simulink model "Tractor_Semitrailer_2023a"  (R2023a)
settings: Solver=VariableStepAuto  StartTime=0.0  StopTime=tmax  FixedStep=dt  RelTol=1e-3  EnableMultiTasking=on
PreLoadFcn:
  | init_vehicle
  | SIMSCAPE_BE_driveline_etrailer_parameters
StartFcn:
  | tic
StopFcn:
  | toc
  | sim_stop_function
undefined symbols (not defined in the file): brake_input, chassis_length, end_val, final_x, final_y, Floor, front_overhang, InputSwitch, L_0f, LD, mass_trailer, massload, pose_t0, sp_t, steer_input, steer_path, steer_ratio, steer_sens, throttle_input, tire_param_drive, tire_param_steer, tire_param_trailer, tire_width, v_0, Vx, wheelbase, X, Y, Z
libraries: sm_lib x367, nesl_utility x273, CommercialVehicleLibrary2G x2, robotalgslib x1, simulink_extras x1
(part 8 of 11)

== system Tractor_Semitrailer_2023a/Tractor_semitrailer /Driver/Control/Simulation end module ==
  x : Inport
  y : Inport  Port=2
  Cast To Boolean : DataTypeConversion  OutDataTypeStr=boolean  SaturateOnIntegerOverflow=off  RndMeth=Floor
  Constant : Constant  Commented=on  Value=end_val
  Constant1 : Constant  Commented=on  Value=end_val
  Constant2 : Constant  Commented=on  Value=v_0
  Constant3 : Constant  Value=final_x
  Constant4 : Constant  Value=final_y
  Constant5 : Constant  Value=0.5
  GreaterThan : RelationalOperator  Commented=on  Operator=<  OutDataTypeStr=boolean  RndMeth=Simplest  InputSameDT=off
  GreaterThan1 : RelationalOperator  Commented=on  Operator=<  OutDataTypeStr=boolean  RndMeth=Simplest  InputSameDT=off
  Less Than : RelationalOperator  Operator=<  OutDataTypeStr=boolean  RndMeth=Simplest  InputSameDT=off
  Scope : Scope
  Sign : Signum  Commented=on
  Sqrt : Sqrt
  Square : Math  Operator=square
  Square1 : Math  Operator=square
  Stop Simulation : Stop  Commented=on
  Stop Simulation1 : Stop
  Sum : Sum
  Sum1 : Sum  Inputs=+-
  Sum2 : Sum  Inputs=+-
  Switch : Switch  Commented=on  Criteria=u2 > Threshold  SaturateOnIntegerOverflow=off  InputSameDT=off
  wires:
  Constant5/1 -> Less Than/2
  Sqrt/1 -> Less Than/1, Scope/1
  Constant4/1 -> Sum2/2
  Sum2/1 -> Square1/1
  Sum1/1 -> Square/1
  Constant3/1 -> Sum1/2
  Sum/1 -> Sqrt/1
  Square1/1 -> Sum/2
  Square/1 -> Sum/1
  Constant/1 -> GreaterThan/2
  x/1 -> Sum1/1
  y/1 -> Sum2/1
  Constant1/1 -> GreaterThan1/2
  Switch/1 -> Stop Simulation/1
  Sign/1 -> Switch/2
  GreaterThan/1 -> Switch/1
  GreaterThan1/1 -> Switch/3
  Constant2/1 -> Sign/1
  Less Than/1 -> Cast To Boolean/1
  Cast To Boolean/1 -> Stop Simulation1/1

== system Tractor_Semitrailer_2023a/Tractor_semitrailer /Semitrailer/Trailer axle 1/Brake//Wheel_bearing ==
  Mdrive : Inport
  Mbrake : Inport  Port=2
  Look-Up Table : Lookup  InputValues=[-5:0.05:5]  Table=-tanh(2*[-5:0.05:5])
  Product1 : Product  InputSameDT=on  SaturateOnIntegerOverflow=on  OutDataTypeStr=Inherit: Same as first input
  Rotational joint around y axis : Subsystem
  Sum : Sum  Inputs=++|
  axle : PMIOPort  Side=Left
  wheel : PMIOPort  Port=2  Side=Right
  omega : Outport  VectorParamsAs1DForOutWhenUnconnected=off
  wires:
  Mbrake/1 -> Product1/1
  Look-Up Table/1 -> Product1/2
  Product1/1 -> Sum/2
  Mdrive/1 -> Sum/1
  Rotational joint around y axis/1(Rotational speed) -> omega/1, Look-Up Table/1
  Sum/1 -> Rotational joint around y axis/1(Torque)
  connections:
  Rotational joint around y axis/LConn1 -- axle/RConn1
  wheel/RConn1 -- Rotational joint around y axis/RConn1

== system Tractor_Semitrailer_2023a/Tractor_semitrailer /Semitrailer/Trailer axle 1/Brake//Wheel_bearing1 ==
  Mdrive : Inport
  Mbrake : Inport  Port=2
  Look-Up Table : Lookup  InputValues=[-5:0.05:5]  Table=-tanh(2*[-5:0.05:5])
  Product1 : Product  InputSameDT=on  SaturateOnIntegerOverflow=on  OutDataTypeStr=Inherit: Same as first input
  Rotational joint around y axis : Subsystem
  Sum : Sum  Inputs=++|
  axle : PMIOPort  Side=Left
  wheel : PMIOPort  Port=2  Side=Right
  omega : Outport  VectorParamsAs1DForOutWhenUnconnected=off
  wires:
  Mbrake/1 -> Product1/1
  Look-Up Table/1 -> Product1/2
  Product1/1 -> Sum/2
  Mdrive/1 -> Sum/1
  Rotational joint around y axis/1(Rotational speed) -> omega/1, Look-Up Table/1
  Sum/1 -> Rotational joint around y axis/1(Torque)
  connections:
  Rotational joint around y axis/LConn1 -- axle/RConn1
  wheel/RConn1 -- Rotational joint around y axis/RConn1

== system Tractor_Semitrailer_2023a/Tractor_semitrailer /Semitrailer/Trailer axle 1/Wheel FL ==
  Bus Creator : BusCreator  Inputs=6
  Bus Creator2 : BusCreator  Inputs=3
  Demux : Demux  Outputs=3
  Demux1 : Demux  Outputs=3
  Geometry Transform : sm_lib/Frames and Transforms/Rigid Transform  TranslationMethod=None  TranslationStandardOffset=0  TranslationStandardOffsetUnits=m  TranslationStandardAxis=+Y  TranslationCartesianOffset=[0 0 0]  TranslationCartesianOffsetUnits=m  TranslationROffset=0  TranslationROffsetUnits=m  TranslationZOffset=0  TranslationZOffsetUnits=m  TranslationThetaOffset=0  TranslationThetaOffsetUnits=deg  RotationMethod=StandardAxis  RotationAngleUnits=deg  RotationStandardAxis=+Z  RotationAngle=sideR*90  RotationArbitraryAxis=[0 0 1]  FollAlignAxisA=+X  BaseAlignAxisA=+Y  FollAlignAxisB=+Y  BaseAlignAxisB=+Z  RotationSequenceAxes=FollowerAxes  RotationSequence=XYX  RotationSequenceAngles=[0 0 0]  RotationSequenceAnglesUnits=deg  RotationMatrix=[1 0 0; 0 1 0; 0 0 1]  Quaternion=[1 0 0 0]
  Inertia : sm_lib/Body Elements/Inertia  InertiaType=Custom  Mass=wheelbody_mass  MassUnits=kg  CenterOfMass=[0 0 0]  CenterOfMassUnits=m  MomentsOfInertia=[Imat(1,1) Imat(2,2) Imat(3,3)]  MomentsOfInertiaUnits=kg*m^2  ProductsOfInertia=[0 0 0]  ProductsOfInertiaUnits=kg*m^2  GraphicType=None  MarkerShape=Inertia  MarkerSize=20  GraphicVisPropType=SimpleVisualProperties  GraphicDiffuseColor=[0.5 0.5 0.5]  GraphicSpecularColor=[0.5 0.5 0.5 1.0]  GraphicAmbientColor=[0.15 0.15 0.15 1.0]  GraphicEmissiveColor=[0.0 0.0 0.0 1.0]  GraphicShininess=75  GraphicOpacity=1.0
  MF Tire FL : sm_lib/Forces and Torques/Magic Formula Tire Force and Torque  TireSide=Left  TireParameters=tire_param  SlipMode=Combined  NumericParameters=[0.1 0.1 0.1 0.1 5.0 1e-4 1e-4 1e-7 1e-7 1e-4 1e-4 0.1 1e-4 1e-4 1e-4 1e-4 1e-4 1e-4 1e-4 1e-4 1e-4]  ScalingCoefficientLMUXMode=FromTireParameters  ScalingCoefficientLMUYMode=FromTireParameters  TireWrenchFrame=ContactFrame  SenseTireForce=on  SenseTireTorque=on  SensePneumaticTrail=off  SenseLongitudinalSlip=off  SenseSaturatedLongitudinalSlip=off  SenseSlipAngle=off  SenseSaturatedSlipAngle=off  SenseTurnSlip=off  SenseRelativeLongitudinalVelocity=off  SenseRelativeLateralVelocity=off  SenseLongitudinalSlipVelocity=off  SenseLateralSlipVelocity=off  SenseYawVelocity=off  SenseCamberAngle=off  SenseSaturatedCamberAngle=off  SenseCamberVelocity=off  SenseSpinVelocity=off  SenseFreeRadius=off  SenseLoadedRadius=off  SenseEffectiveRollingRadius=off  SenseLongitudinalFrictionCoefficient=off  SenseLateralFrictionCoefficient=off  SenseContactBaseRotation=off  SenseContactBaseTranslation=off  SenseContactFollowerRotation=off  SenseContactFollowerTranslation=off
  PS-Simulink Converter : nesl_utility/PS-Simulink Converter  PhysicalDomain=network_engine_domain  SubClassName=ps_output  LeftPortType=input  RightPortType=output  PseudoPeriodic=off  Frequencies=[]  VectorFormat=inherit  Unit=inherit  AffineConversion=off
  PS-Simulink Converter1 : nesl_utility/PS-Simulink Converter  PhysicalDomain=network_engine_domain  SubClassName=ps_output  LeftPortType=input  RightPortType=output  PseudoPeriodic=off  Frequencies=[]  VectorFormat=inherit  Unit=inherit  AffineConversion=off
  PS-Simulink Converter{2..11} (10 alike) : nesl_utility/PS-Simulink Converter  PhysicalDomain=network_engine_domain  SubClassName=ps_output  LeftPortType=input  RightPortType=output  PseudoPeriodic=off  Frequencies=[]  VectorFormat=1-D array  Unit=1  AffineConversion=off
  Reshape : Reshape
  Rigid Transform : sm_lib/Frames and Transforms/Rigid Transform  TranslationMethod=StandardAxis  TranslationStandardOffset=tire_width/2  TranslationStandardOffsetUnits=m  TranslationStandardAxis=+Z  TranslationCartesianOffset=[0 0 0]  TranslationCartesianOffsetUnits=m  TranslationROffset=0  TranslationROffsetUnits=m  TranslationZOffset=0  TranslationZOffsetUnits=m  TranslationThetaOffset=0  TranslationThetaOffsetUnits=deg  RotationMethod=None  RotationAngleUnits=deg  RotationStandardAxis=+Z  RotationAngle=0.0  RotationArbitraryAxis=[0 0 1]  FollAlignAxisA=+X  BaseAlignAxisA=+Y  FollAlignAxisB=+Y  BaseAlignAxisB=+Z  RotationSequenceAxes=FollowerAxes  RotationSequence=XYX  RotationSequenceAngles=[0 0 0]  RotationSequenceAnglesUnits=deg  RotationMatrix=[1 0 0; 0 1 0; 0 0 1]  Quaternion=[1 0 0 0]
  Rim+Tire : sm_lib/Body Elements/File Solid  ExtGeomFileName=wheel.STP  UnitType=Custom  ExtGeomFileUnits=mm  StepReaderType=HEX  ExportConvexHullGeometry=off  InertiaType=Custom  Mass=0  MassUnits=kg  CenterOfMass=[0 0 0]  CenterOfMassUnits=m  MomentsOfInertia=[0 0 0]  MomentsOfInertiaUnits=kg*m^2  ProductsOfInertia=[0 0 0]  ProductsOfInertiaUnits=kg*m^2  BasedOnType=Density  Density=1000  DensityUnits=kg/(m^3)  DoExposeReferenceFrame=on  SerializedFrames=<Frames/>  GraphicType=FromGeometry  MarkerShape=Sphere  MarkerSize=10  GraphicVisPropType=SimpleVisualProperties  GraphicDiffuseColor=[0.8 0.8 0.8]  GraphicSpecularColor=[0.5 0.5 0.5 1.0]  GraphicAmbientColor=[0.15 0.15 0.15 1.0]  GraphicEmissiveColor=[0.0 0.0 0.0 1.0]  GraphicShininess=75  GraphicOpacity=1.0
  Rotation Axis Transform : sm_lib/Frames and Transforms/Rigid Transform  TranslationMethod=None  TranslationStandardOffset=0  TranslationStandardOffsetUnits=m  TranslationStandardAxis=+Z  TranslationCartesianOffset=[0 0 0]  TranslationCartesianOffsetUnits=m  TranslationROffset=0  TranslationROffsetUnits=m  TranslationZOffset=0  TranslationZOffsetUnits=m  TranslationThetaOffset=0  TranslationThetaOffsetUnits=deg  RotationMethod=AlignedAxes  RotationAngleUnits=deg  RotationStandardAxis=-X  RotationAngle=0  RotationArbitraryAxis=[0 0 1]  FollAlignAxisA=+X  BaseAlignAxisA=+X  FollAlignAxisB=+Z  BaseAlignAxisB=+Y  RotationSequenceAxes=FollowerAxes  RotationSequence=XYX  RotationSequenceAngles=[0 0 0]  RotationSequenceAnglesUnits=deg  RotationMatrix=[1 0 0; 0 1 0; 0 0 1]  Quaternion=[1 0 0 0]
  Terminator{,1..6} (7 alike) : Terminator
  Transform Sensor-LocalBodyCS : sm_lib/Frames and Transforms/Transform Sensor  MeasurementFrame=NonRotatingFollower  RotationSequence=XYX  SenseAngle=off  SenseAxis=off  SenseQ=off  SenseR=off  SenseRotationSequence=off  SenseOmegaX=on  SenseOmegaY=on  SenseOmegaZ=on  SenseQDot=off  SenseRDot=off  SenseRotationSequenceDot=off  SenseAlphaX=off  SenseAlphaY=off  SenseAlphaZ=off  SenseQDDot=off  SenseRDDot=off  SenseX=off  SenseY=off  SenseZ=off  SenseRad=off  SenseAzim=off  SenseDist=off  SenseInc=off  SenseXDot=on  SenseYDot=on  SenseZDot=on  SenseRadDot=off  SenseAzimDot=off  SenseDistDot=off  SenseIncDot=off  SenseXDDot=off  SenseYDDot=off  SenseZDDot=off  SenseRadDDot=off  SenseAzimDDot=off  SenseDistDDot=off  SenseIncDDot=off
  Transform Sensor-WorldCS : sm_lib/Frames and Transforms/Transform Sensor  MeasurementFrame=World  RotationSequence=XYX  SenseAngle=off  SenseAxis=off  SenseQ=off  SenseR=on  SenseRotationSequence=off  SenseOmegaX=off  SenseOmegaY=off  SenseOmegaZ=off  SenseQDot=off  SenseRDot=off  SenseRotationSequenceDot=off  SenseAlphaX=off  SenseAlphaY=off  SenseAlphaZ=off  SenseQDDot=off  SenseRDDot=off  SenseX=on  SenseY=on  SenseZ=on  SenseRad=off  SenseAzim=off  SenseDist=off  SenseInc=off  SenseXDot=off  SenseYDot=off  SenseZDot=off  SenseRadDot=off  SenseAzimDot=off  SenseDistDot=off  SenseIncDot=off  SenseXDDot=off  SenseYDDot=off  SenseZDDot=off  SenseRadDDot=off  SenseAzimDDot=off  SenseDistDDot=off  SenseIncDDot=off
  World Frame : sm_lib/Frames and Transforms/World Frame
  "Wheel " : PMIOPort  Side=Left
  Ground : PMIOPort  Port=2  Side=Left
  Tire Foces : Outport
  Tire Position : Outport  Port=2
  wires:
  PS-Simulink Converter/1 -> Demux/1
  Demux/2 -> Bus Creator/2  "Lateral: Fy"
  Bus Creator/1 -> Tire Foces/1
  Demux/3 -> Bus Creator/3  "Normal: Fz"
  PS-Simulink Converter1/1 -> Demux1/1
  Demux1/2 -> Bus Creator/5  "Rolling Resistance: My"
  Demux1/3 -> Bus Creator/6  "Aligning: Mz"
  Demux1/1 -> Bus Creator/4  "Overturning: Mx"
  Demux/1 -> Bus Creator/1  "Longitudinal: Fx"
  PS-Simulink Converter6/1 -> Terminator1/1  "wx"
  PS-Simulink Converter10/1 -> Terminator5/1  "vy"
  PS-Simulink Converter8/1 -> Terminator3/1  "wz"
  PS-Simulink Converter2/1 -> Reshape/1
  PS-Simulink Converter9/1 -> Terminator4/1  "vx"
  PS-Simulink Converter5/1 -> Bus Creator2/3  "z"
  Bus Creator2/1 -> Tire Position/1
  PS-Simulink Converter7/1 -> Terminator2/1  "wy"
  Reshape/1 -> Terminator/1  "R"
  PS-Simulink Converter3/1 -> Bus Creator2/1  "x"
  PS-Simulink Converter4/1 -> Bus Creator2/2  "y"
  PS-Simulink Converter11/1 -> Terminator6/1  "vz"
  connections:
  PS-Simulink Converter1/LConn1 -- MF Tire FL/RConn3
  PS-Simulink Converter/LConn1 -- MF Tire FL/RConn2
  Ground/RConn1 -- MF Tire FL/LConn1
  Transform Sensor-LocalBodyCS/RConn1 -- Rotation Axis Transform/RConn1 -- "Wheel "/RConn1 -- MF Tire FL/RConn1 -- Rigid Transform/LConn1
  Rim+Tire/RConn1 -- Geometry Transform/RConn1
  Geometry Transform/LConn1 -- Inertia/RConn1 -- Rotation Axis Transform/LConn1
  Transform Sensor-LocalBodyCS/LConn1 -- World Frame/RConn1 -- Transform Sensor-WorldCS/LConn1
  Transform Sensor-WorldCS/RConn1 -- Rigid Transform/RConn1
  Transform Sensor-WorldCS/RConn4 -- PS-Simulink Converter4/LConn1
  Transform Sensor-LocalBodyCS/RConn7 -- PS-Simulink Converter11/LConn1
  Transform Sensor-LocalBodyCS/RConn5 -- PS-Simulink Converter9/LConn1
  Transform Sensor-WorldCS/RConn2 -- PS-Simulink Converter2/LConn1
  Transform Sensor-WorldCS/RConn5 -- PS-Simulink Converter5/LConn1
  Transform Sensor-LocalBodyCS/RConn2 -- PS-Simulink Converter6/LConn1
  Transform Sensor-WorldCS/RConn3 -- PS-Simulink Converter3/LConn1
  Transform Sensor-LocalBodyCS/RConn3 -- PS-Simulink Converter7/LConn1
  Transform Sensor-LocalBodyCS/RConn4 -- PS-Simulink Converter8/LConn1
  Transform Sensor-LocalBodyCS/RConn6 -- PS-Simulink Converter10/LConn1

== system Tractor_Semitrailer_2023a/Tractor_semitrailer /Semitrailer/Trailer axle 1/Wheel FR ==
  Bus Creator : BusCreator  Inputs=6
  Bus Creator2 : BusCreator  Inputs=3
  Demux : Demux  Outputs=3
  Demux1 : Demux  Outputs=3
  Geometry Transform : sm_lib/Frames and Transforms/Rigid Transform  TranslationMethod=None  TranslationStandardOffset=0  TranslationStandardOffsetUnits=m  TranslationStandardAxis=+Y  TranslationCartesianOffset=[0 0 0]  TranslationCartesianOffsetUnits=m  TranslationROffset=0  TranslationROffsetUnits=m  TranslationZOffset=0  TranslationZOffsetUnits=m  TranslationThetaOffset=0  TranslationThetaOffsetUnits=deg  RotationMethod=StandardAxis  RotationAngleUnits=deg  RotationStandardAxis=+Z  RotationAngle=sideL*90  RotationArbitraryAxis=[0 0 1]  FollAlignAxisA=+X  BaseAlignAxisA=+Y  FollAlignAxisB=+Y  BaseAlignAxisB=+Z  RotationSequenceAxes=FollowerAxes  RotationSequence=XYX  RotationSequenceAngles=[0 0 0]  RotationSequenceAnglesUnits=deg  RotationMatrix=[1 0 0; 0 1 0; 0 0 1]  Quaternion=[1 0 0 0]
  Inertia : sm_lib/Body Elements/Inertia  InertiaType=Custom  Mass=wheelbody_mass  MassUnits=kg  CenterOfMass=[0 0 0]  CenterOfMassUnits=m  MomentsOfInertia=[Imat(1,1) Imat(2,2) Imat(3,3)]  MomentsOfInertiaUnits=kg*m^2  ProductsOfInertia=[0 0 0]  ProductsOfInertiaUnits=kg*m^2  GraphicType=None  MarkerShape=Inertia  MarkerSize=20  GraphicVisPropType=SimpleVisualProperties  GraphicDiffuseColor=[0.5 0.5 0.5]  GraphicSpecularColor=[0.5 0.5 0.5 1.0]  GraphicAmbientColor=[0.15 0.15 0.15 1.0]  GraphicEmissiveColor=[0.0 0.0 0.0 1.0]  GraphicShininess=75  GraphicOpacity=1.0
  MF Tire FL : sm_lib/Forces and Torques/Magic Formula Tire Force and Torque  TireSide=Right  TireParameters=tire_param  SlipMode=Combined  NumericParameters=[0.1 0.1 0.1 0.1 5.0 1e-4 1e-4 1e-7 1e-7 1e-4 1e-4 0.1 1e-4 1e-4 1e-4 1e-4 1e-4 1e-4 1e-4 1e-4 1e-4]  ScalingCoefficientLMUXMode=FromTireParameters  ScalingCoefficientLMUYMode=FromTireParameters  TireWrenchFrame=ContactFrame  SenseTireForce=on  SenseTireTorque=on  SensePneumaticTrail=off  SenseLongitudinalSlip=off  SenseSaturatedLongitudinalSlip=off  SenseSlipAngle=off  SenseSaturatedSlipAngle=off  SenseTurnSlip=off  SenseRelativeLongitudinalVelocity=off  SenseRelativeLateralVelocity=off  SenseLongitudinalSlipVelocity=off  SenseLateralSlipVelocity=off  SenseYawVelocity=off  SenseCamberAngle=off  SenseSaturatedCamberAngle=off  SenseCamberVelocity=off  SenseSpinVelocity=off  SenseFreeRadius=off  SenseLoadedRadius=off  SenseEffectiveRollingRadius=off  SenseLongitudinalFrictionCoefficient=off  SenseLateralFrictionCoefficient=off  SenseContactBaseRotation=off  SenseContactBaseTranslation=off  SenseContactFollowerRotation=off  SenseContactFollowerTranslation=off
  PS-Simulink Converter : nesl_utility/PS-Simulink Converter  PhysicalDomain=network_engine_domain  SubClassName=ps_output  LeftPortType=input  RightPortType=output  PseudoPeriodic=off  Frequencies=[]  VectorFormat=inherit  Unit=inherit  AffineConversion=off
  PS-Simulink Converter1 : nesl_utility/PS-Simulink Converter  PhysicalDomain=network_engine_domain  SubClassName=ps_output  LeftPortType=input  RightPortType=output  PseudoPeriodic=off  Frequencies=[]  VectorFormat=inherit  Unit=inherit  AffineConversion=off
  PS-Simulink Converter{2..11} (10 alike) : nesl_utility/PS-Simulink Converter  PhysicalDomain=network_engine_domain  SubClassName=ps_output  LeftPortType=input  RightPortType=output  PseudoPeriodic=off  Frequencies=[]  VectorFormat=1-D array  Unit=1  AffineConversion=off
  Reshape : Reshape
  Rigid Transform : sm_lib/Frames and Transforms/Rigid Transform  TranslationMethod=StandardAxis  TranslationStandardOffset=tire_width/2  TranslationStandardOffsetUnits=m  TranslationStandardAxis=-Z  TranslationCartesianOffset=[0 0 0]  TranslationCartesianOffsetUnits=m  TranslationROffset=0  TranslationROffsetUnits=m  TranslationZOffset=0  TranslationZOffsetUnits=m  TranslationThetaOffset=0  TranslationThetaOffsetUnits=deg  RotationMethod=None  RotationAngleUnits=deg  RotationStandardAxis=+Z  RotationAngle=0.0  RotationArbitraryAxis=[0 0 1]  FollAlignAxisA=+X  BaseAlignAxisA=+Y  FollAlignAxisB=+Y  BaseAlignAxisB=+Z  RotationSequenceAxes=FollowerAxes  RotationSequence=XYX  RotationSequenceAngles=[0 0 0]  RotationSequenceAnglesUnits=deg  RotationMatrix=[1 0 0; 0 1 0; 0 0 1]  Quaternion=[1 0 0 0]
  Rim+Tire : sm_lib/Body Elements/File Solid  ExtGeomFileName=wheel.STP  UnitType=Custom  ExtGeomFileUnits=mm  StepReaderType=HEX  ExportConvexHullGeometry=off  InertiaType=Custom  Mass=0  MassUnits=kg  CenterOfMass=[0 0 0]  CenterOfMassUnits=m  MomentsOfInertia=[0 0 0]  MomentsOfInertiaUnits=kg*m^2  ProductsOfInertia=[0 0 0]  ProductsOfInertiaUnits=kg*m^2  BasedOnType=Density  Density=1000  DensityUnits=kg/(m^3)  DoExposeReferenceFrame=on  SerializedFrames=<Frames/>  GraphicType=FromGeometry  MarkerShape=Sphere  MarkerSize=10  GraphicVisPropType=SimpleVisualProperties  GraphicDiffuseColor=[0.8 0.8 0.8]  GraphicSpecularColor=[0.5 0.5 0.5 1.0]  GraphicAmbientColor=[0.15 0.15 0.15 1.0]  GraphicEmissiveColor=[0.0 0.0 0.0 1.0]  GraphicShininess=75  GraphicOpacity=1.0
  Rotation Axis Transform : sm_lib/Frames and Transforms/Rigid Transform  TranslationMethod=None  TranslationStandardOffset=0  TranslationStandardOffsetUnits=m  TranslationStandardAxis=+Z  TranslationCartesianOffset=[0 0 0]  TranslationCartesianOffsetUnits=m  TranslationROffset=0  TranslationROffsetUnits=m  TranslationZOffset=0  TranslationZOffsetUnits=m  TranslationThetaOffset=0  TranslationThetaOffsetUnits=deg  RotationMethod=AlignedAxes  RotationAngleUnits=deg  RotationStandardAxis=-X  RotationAngle=0  RotationArbitraryAxis=[0 0 1]  FollAlignAxisA=+X  BaseAlignAxisA=+X  FollAlignAxisB=+Z  BaseAlignAxisB=+Y  RotationSequenceAxes=FollowerAxes  RotationSequence=XYX  RotationSequenceAngles=[0 0 0]  RotationSequenceAnglesUnits=deg  RotationMatrix=[1 0 0; 0 1 0; 0 0 1]  Quaternion=[1 0 0 0]
  Terminator{,1..6} (7 alike) : Terminator
  Transform Sensor-LocalBodyCS : sm_lib/Frames and Transforms/Transform Sensor  MeasurementFrame=NonRotatingFollower  RotationSequence=XYX  SenseAngle=off  SenseAxis=off  SenseQ=off  SenseR=off  SenseRotationSequence=off  SenseOmegaX=on  SenseOmegaY=on  SenseOmegaZ=on  SenseQDot=off  SenseRDot=off  SenseRotationSequenceDot=off  SenseAlphaX=off  SenseAlphaY=off  SenseAlphaZ=off  SenseQDDot=off  SenseRDDot=off  SenseX=off  SenseY=off  SenseZ=off  SenseRad=off  SenseAzim=off  SenseDist=off  SenseInc=off  SenseXDot=on  SenseYDot=on  SenseZDot=on  SenseRadDot=off  SenseAzimDot=off  SenseDistDot=off  SenseIncDot=off  SenseXDDot=off  SenseYDDot=off  SenseZDDot=off  SenseRadDDot=off  SenseAzimDDot=off  SenseDistDDot=off  SenseIncDDot=off
  Transform Sensor-WorldCS : sm_lib/Frames and Transforms/Transform Sensor  MeasurementFrame=World  RotationSequence=XYX  SenseAngle=off  SenseAxis=off  SenseQ=off  SenseR=on  SenseRotationSequence=off  SenseOmegaX=off  SenseOmegaY=off  SenseOmegaZ=off  SenseQDot=off  SenseRDot=off  SenseRotationSequenceDot=off  SenseAlphaX=off  SenseAlphaY=off  SenseAlphaZ=off  SenseQDDot=off  SenseRDDot=off  SenseX=on  SenseY=on  SenseZ=on  SenseRad=off  SenseAzim=off  SenseDist=off  SenseInc=off  SenseXDot=off  SenseYDot=off  SenseZDot=off  SenseRadDot=off  SenseAzimDot=off  SenseDistDot=off  SenseIncDot=off  SenseXDDot=off  SenseYDDot=off  SenseZDDot=off  SenseRadDDot=off  SenseAzimDDot=off  SenseDistDDot=off  SenseIncDDot=off
  World Frame : sm_lib/Frames and Transforms/World Frame
  "Wheel " : PMIOPort  Side=Left
  Ground : PMIOPort  Port=2  Side=Left
  Tire Foces : Outport
  Tire Position : Outport  Port=2
  wires:
  PS-Simulink Converter/1 -> Demux/1
  Demux/2 -> Bus Creator/2  "Lateral: Fy"
  Bus Creator/1 -> Tire Foces/1
  Demux/3 -> Bus Creator/3  "Normal: Fz"
  PS-Simulink Converter1/1 -> Demux1/1
  Demux1/2 -> Bus Creator/5  "Rolling Resistance: My"
  Demux1/3 -> Bus Creator/6  "Aligning: Mz"
  Demux1/1 -> Bus Creator/4  "Overturning: Mx"
  Demux/1 -> Bus Creator/1  "Longitudinal: Fx"
  PS-Simulink Converter6/1 -> Terminator1/1  "wx"
  PS-Simulink Converter10/1 -> Terminator5/1  "vy"
  PS-Simulink Converter8/1 -> Terminator3/1  "wz"
  PS-Simulink Converter2/1 -> Reshape/1
  PS-Simulink Converter9/1 -> Terminator4/1  "vx"
  PS-Simulink Converter5/1 -> Bus Creator2/3  "z"
  Bus Creator2/1 -> Tire Position/1
  PS-Simulink Converter7/1 -> Terminator2/1  "wy"
  Reshape/1 -> Terminator/1  "R"
  PS-Simulink Converter3/1 -> Bus Creator2/1  "x"
  PS-Simulink Converter4/1 -> Bus Creator2/2  "y"
  PS-Simulink Converter11/1 -> Terminator6/1  "vz"
  connections:
  PS-Simulink Converter1/LConn1 -- MF Tire FL/RConn3
  PS-Simulink Converter/LConn1 -- MF Tire FL/RConn2
  Ground/RConn1 -- MF Tire FL/LConn1
  Transform Sensor-LocalBodyCS/RConn1 -- "Wheel "/RConn1 -- Rotation Axis Transform/RConn1 -- MF Tire FL/RConn1 -- Rigid Transform/LConn1
  Rim+Tire/RConn1 -- Geometry Transform/RConn1
  Geometry Transform/LConn1 -- Inertia/RConn1 -- Rotation Axis Transform/LConn1
  Transform Sensor-LocalBodyCS/LConn1 -- World Frame/RConn1 -- Transform Sensor-WorldCS/LConn1
  Transform Sensor-WorldCS/RConn1 -- Rigid Transform/RConn1
  Transform Sensor-WorldCS/RConn4 -- PS-Simulink Converter4/LConn1
  Transform Sensor-LocalBodyCS/RConn7 -- PS-Simulink Converter11/LConn1
  Transform Sensor-LocalBodyCS/RConn5 -- PS-Simulink Converter9/LConn1
  Transform Sensor-WorldCS/RConn2 -- PS-Simulink Converter2/LConn1
  Transform Sensor-WorldCS/RConn5 -- PS-Simulink Converter5/LConn1
  Transform Sensor-LocalBodyCS/RConn2 -- PS-Simulink Converter6/LConn1
  Transform Sensor-WorldCS/RConn3 -- PS-Simulink Converter3/LConn1
  Transform Sensor-LocalBodyCS/RConn3 -- PS-Simulink Converter7/LConn1
  Transform Sensor-LocalBodyCS/RConn4 -- PS-Simulink Converter8/LConn1
  Transform Sensor-LocalBodyCS/RConn6 -- PS-Simulink Converter10/LConn1

== system Tractor_Semitrailer_2023a/Tractor_semitrailer /Semitrailer/Trailer axle 2/Brake//Wheel_bearing ==
  Mdrive : Inport
  Mbrake : Inport  Port=2
  Look-Up Table : Lookup  InputValues=[-5:0.05:5]  Table=-tanh(2*[-5:0.05:5])
  Product1 : Product  InputSameDT=on  SaturateOnIntegerOverflow=on  OutDataTypeStr=Inherit: Same as first input
  Rotational joint around y axis : Subsystem
  Sum : Sum  Inputs=++|
  axle : PMIOPort  Side=Left
  wheel : PMIOPort  Port=2  Side=Right
  omega : Outport  VectorParamsAs1DForOutWhenUnconnected=off
  wires:
  Mbrake/1 -> Product1/1
  Look-Up Table/1 -> Product1/2
  Product1/1 -> Sum/2
  Mdrive/1 -> Sum/1
  Rotational joint around y axis/1(Rotational speed) -> omega/1, Look-Up Table/1
  Sum/1 -> Rotational joint around y axis/1(Torque)
  connections:
  Rotational joint around y axis/LConn1 -- axle/RConn1
  wheel/RConn1 -- Rotational joint around y axis/RConn1

== system Tractor_Semitrailer_2023a/Tractor_semitrailer /Semitrailer/Trailer axle 2/Brake//Wheel_bearing1 ==
  Mdrive : Inport
  Mbrake : Inport  Port=2
  Look-Up Table : Lookup  InputValues=[-5:0.05:5]  Table=-tanh(2*[-5:0.05:5])
  Product1 : Product  InputSameDT=on  SaturateOnIntegerOverflow=on  OutDataTypeStr=Inherit: Same as first input
  Rotational joint around y axis : Subsystem
  Sum : Sum  Inputs=++|
  axle : PMIOPort  Side=Left
  wheel : PMIOPort  Port=2  Side=Right
  omega : Outport  VectorParamsAs1DForOutWhenUnconnected=off
  wires:
  Mbrake/1 -> Product1/1
  Look-Up Table/1 -> Product1/2
  Product1/1 -> Sum/2
  Mdrive/1 -> Sum/1
  Rotational joint around y axis/1(Rotational speed) -> omega/1, Look-Up Table/1
  Sum/1 -> Rotational joint around y axis/1(Torque)
  connections:
  Rotational joint around y axis/LConn1 -- axle/RConn1
  wheel/RConn1 -- Rotational joint around y axis/RConn1

== system Tractor_Semitrailer_2023a/Tractor_semitrailer /Semitrailer/Trailer axle 2/Wheel FL ==
  Bus Creator : BusCreator  Inputs=6
  Bus Creator2 : BusCreator  Inputs=3
  Demux : Demux  Outputs=3
  Demux1 : Demux  Outputs=3
  Geometry Transform : sm_lib/Frames and Transforms/Rigid Transform  TranslationMethod=None  TranslationStandardOffset=0  TranslationStandardOffsetUnits=m  TranslationStandardAxis=+Y  TranslationCartesianOffset=[0 0 0]  TranslationCartesianOffsetUnits=m  TranslationROffset=0  TranslationROffsetUnits=m  TranslationZOffset=0  TranslationZOffsetUnits=m  TranslationThetaOffset=0  TranslationThetaOffsetUnits=deg  RotationMethod=StandardAxis  RotationAngleUnits=deg  RotationStandardAxis=+Z  RotationAngle=sideR*90  RotationArbitraryAxis=[0 0 1]  FollAlignAxisA=+X  BaseAlignAxisA=+Y  FollAlignAxisB=+Y  BaseAlignAxisB=+Z  RotationSequenceAxes=FollowerAxes  RotationSequence=XYX  RotationSequenceAngles=[0 0 0]  RotationSequenceAnglesUnits=deg  RotationMatrix=[1 0 0; 0 1 0; 0 0 1]  Quaternion=[1 0 0 0]
  Inertia : sm_lib/Body Elements/Inertia  InertiaType=Custom  Mass=wheelbody_mass  MassUnits=kg  CenterOfMass=[0 0 0]  CenterOfMassUnits=m  MomentsOfInertia=[Imat(1,1) Imat(2,2) Imat(3,3)]  MomentsOfInertiaUnits=kg*m^2  ProductsOfInertia=[0 0 0]  ProductsOfInertiaUnits=kg*m^2  GraphicType=None  MarkerShape=Inertia  MarkerSize=20  GraphicVisPropType=SimpleVisualProperties  GraphicDiffuseColor=[0.5 0.5 0.5]  GraphicSpecularColor=[0.5 0.5 0.5 1.0]  GraphicAmbientColor=[0.15 0.15 0.15 1.0]  GraphicEmissiveColor=[0.0 0.0 0.0 1.0]  GraphicShininess=75  GraphicOpacity=1.0
  MF Tire FL : sm_lib/Forces and Torques/Magic Formula Tire Force and Torque  TireSide=Left  TireParameters=tire_param  SlipMode=Combined  NumericParameters=[0.1 0.1 0.1 0.1 5.0 1e-4 1e-4 1e-7 1e-7 1e-4 1e-4 0.1 1e-4 1e-4 1e-4 1e-4 1e-4 1e-4 1e-4 1e-4 1e-4]  ScalingCoefficientLMUXMode=FromTireParameters  ScalingCoefficientLMUYMode=FromTireParameters  TireWrenchFrame=ContactFrame  SenseTireForce=on  SenseTireTorque=on  SensePneumaticTrail=off  SenseLongitudinalSlip=off  SenseSaturatedLongitudinalSlip=off  SenseSlipAngle=off  SenseSaturatedSlipAngle=off  SenseTurnSlip=off  SenseRelativeLongitudinalVelocity=off  SenseRelativeLateralVelocity=off  SenseLongitudinalSlipVelocity=off  SenseLateralSlipVelocity=off  SenseYawVelocity=off  SenseCamberAngle=off  SenseSaturatedCamberAngle=off  SenseCamberVelocity=off  SenseSpinVelocity=off  SenseFreeRadius=off  SenseLoadedRadius=off  SenseEffectiveRollingRadius=off  SenseLongitudinalFrictionCoefficient=off  SenseLateralFrictionCoefficient=off  SenseContactBaseRotation=off  SenseContactBaseTranslation=off  SenseContactFollowerRotation=off  SenseContactFollowerTranslation=off
  PS-Simulink Converter : nesl_utility/PS-Simulink Converter  PhysicalDomain=network_engine_domain  SubClassName=ps_output  LeftPortType=input  RightPortType=output  PseudoPeriodic=off  Frequencies=[]  VectorFormat=inherit  Unit=inherit  AffineConversion=off
  PS-Simulink Converter1 : nesl_utility/PS-Simulink Converter  PhysicalDomain=network_engine_domain  SubClassName=ps_output  LeftPortType=input  RightPortType=output  PseudoPeriodic=off  Frequencies=[]  VectorFormat=inherit  Unit=inherit  AffineConversion=off
  PS-Simulink Converter{2..11} (10 alike) : nesl_utility/PS-Simulink Converter  PhysicalDomain=network_engine_domain  SubClassName=ps_output  LeftPortType=input  RightPortType=output  PseudoPeriodic=off  Frequencies=[]  VectorFormat=1-D array  Unit=1  AffineConversion=off
  Reshape : Reshape
  Rigid Transform : sm_lib/Frames and Transforms/Rigid Transform  TranslationMethod=StandardAxis  TranslationStandardOffset=tire_width/2  TranslationStandardOffsetUnits=m  TranslationStandardAxis=+Z  TranslationCartesianOffset=[0 0 0]  TranslationCartesianOffsetUnits=m  TranslationROffset=0  TranslationROffsetUnits=m  TranslationZOffset=0  TranslationZOffsetUnits=m  TranslationThetaOffset=0  TranslationThetaOffsetUnits=deg  RotationMethod=None  RotationAngleUnits=deg  RotationStandardAxis=+Z  RotationAngle=0.0  RotationArbitraryAxis=[0 0 1]  FollAlignAxisA=+X  BaseAlignAxisA=+Y  FollAlignAxisB=+Y  BaseAlignAxisB=+Z  RotationSequenceAxes=FollowerAxes  RotationSequence=XYX  RotationSequenceAngles=[0 0 0]  RotationSequenceAnglesUnits=deg  RotationMatrix=[1 0 0; 0 1 0; 0 0 1]  Quaternion=[1 0 0 0]
  Rim+Tire : sm_lib/Body Elements/File Solid  ExtGeomFileName=wheel.STP  UnitType=Custom  ExtGeomFileUnits=mm  StepReaderType=HEX  ExportConvexHullGeometry=off  InertiaType=Custom  Mass=0  MassUnits=kg  CenterOfMass=[0 0 0]  CenterOfMassUnits=m  MomentsOfInertia=[0 0 0]  MomentsOfInertiaUnits=kg*m^2  ProductsOfInertia=[0 0 0]  ProductsOfInertiaUnits=kg*m^2  BasedOnType=Density  Density=1000  DensityUnits=kg/(m^3)  DoExposeReferenceFrame=on  SerializedFrames=<Frames/>  GraphicType=FromGeometry  MarkerShape=Sphere  MarkerSize=10  GraphicVisPropType=SimpleVisualProperties  GraphicDiffuseColor=[0.8 0.8 0.8]  GraphicSpecularColor=[0.5 0.5 0.5 1.0]  GraphicAmbientColor=[0.15 0.15 0.15 1.0]  GraphicEmissiveColor=[0.0 0.0 0.0 1.0]  GraphicShininess=75  GraphicOpacity=1.0
  Rotation Axis Transform : sm_lib/Frames and Transforms/Rigid Transform  TranslationMethod=None  TranslationStandardOffset=0  TranslationStandardOffsetUnits=m  TranslationStandardAxis=+Z  TranslationCartesianOffset=[0 0 0]  TranslationCartesianOffsetUnits=m  TranslationROffset=0  TranslationROffsetUnits=m  TranslationZOffset=0  TranslationZOffsetUnits=m  TranslationThetaOffset=0  TranslationThetaOffsetUnits=deg  RotationMethod=AlignedAxes  RotationAngleUnits=deg  RotationStandardAxis=-X  RotationAngle=0  RotationArbitraryAxis=[0 0 1]  FollAlignAxisA=+X  BaseAlignAxisA=+X  FollAlignAxisB=+Z  BaseAlignAxisB=+Y  RotationSequenceAxes=FollowerAxes  RotationSequence=XYX  RotationSequenceAngles=[0 0 0]  RotationSequenceAnglesUnits=deg  RotationMatrix=[1 0 0; 0 1 0; 0 0 1]  Quaternion=[1 0 0 0]
  Terminator{,1..6} (7 alike) : Terminator
  Transform Sensor-LocalBodyCS : sm_lib/Frames and Transforms/Transform Sensor  MeasurementFrame=NonRotatingFollower  RotationSequence=XYX  SenseAngle=off  SenseAxis=off  SenseQ=off  SenseR=off  SenseRotationSequence=off  SenseOmegaX=on  SenseOmegaY=on  SenseOmegaZ=on  SenseQDot=off  SenseRDot=off  SenseRotationSequenceDot=off  SenseAlphaX=off  SenseAlphaY=off  SenseAlphaZ=off  SenseQDDot=off  SenseRDDot=off  SenseX=off  SenseY=off  SenseZ=off  SenseRad=off  SenseAzim=off  SenseDist=off  SenseInc=off  SenseXDot=on  SenseYDot=on  SenseZDot=on  SenseRadDot=off  SenseAzimDot=off  SenseDistDot=off  SenseIncDot=off  SenseXDDot=off  SenseYDDot=off  SenseZDDot=off  SenseRadDDot=off  SenseAzimDDot=off  SenseDistDDot=off  SenseIncDDot=off
  Transform Sensor-WorldCS : sm_lib/Frames and Transforms/Transform Sensor  MeasurementFrame=World  RotationSequence=XYX  SenseAngle=off  SenseAxis=off  SenseQ=off  SenseR=on  SenseRotationSequence=off  SenseOmegaX=off  SenseOmegaY=off  SenseOmegaZ=off  SenseQDot=off  SenseRDot=off  SenseRotationSequenceDot=off  SenseAlphaX=off  SenseAlphaY=off  SenseAlphaZ=off  SenseQDDot=off  SenseRDDot=off  SenseX=on  SenseY=on  SenseZ=on  SenseRad=off  SenseAzim=off  SenseDist=off  SenseInc=off  SenseXDot=off  SenseYDot=off  SenseZDot=off  SenseRadDot=off  SenseAzimDot=off  SenseDistDot=off  SenseIncDot=off  SenseXDDot=off  SenseYDDot=off  SenseZDDot=off  SenseRadDDot=off  SenseAzimDDot=off  SenseDistDDot=off  SenseIncDDot=off
  World Frame : sm_lib/Frames and Transforms/World Frame
  "Wheel " : PMIOPort  Side=Left
  Ground : PMIOPort  Port=2  Side=Left
  Tire Foces : Outport
  Tire Position : Outport  Port=2
  wires:
  PS-Simulink Converter/1 -> Demux/1
  Demux/2 -> Bus Creator/2  "Lateral: Fy"
  Bus Creator/1 -> Tire Foces/1
  Demux/3 -> Bus Creator/3  "Normal: Fz"
  PS-Simulink Converter1/1 -> Demux1/1
  Demux1/2 -> Bus Creator/5  "Rolling Resistance: My"
  Demux1/3 -> Bus Creator/6  "Aligning: Mz"
  Demux1/1 -> Bus Creator/4  "Overturning: Mx"
  Demux/1 -> Bus Creator/1  "Longitudinal: Fx"
  PS-Simulink Converter6/1 -> Terminator1/1  "wx"
  PS-Simulink Converter10/1 -> Terminator5/1  "vy"
  PS-Simulink Converter8/1 -> Terminator3/1  "wz"
  PS-Simulink Converter2/1 -> Reshape/1
  PS-Simulink Converter9/1 -> Terminator4/1  "vx"
  PS-Simulink Converter5/1 -> Bus Creator2/3  "z"
  Bus Creator2/1 -> Tire Position/1
  PS-Simulink Converter7/1 -> Terminator2/1  "wy"
  Reshape/1 -> Terminator/1  "R"
  PS-Simulink Converter3/1 -> Bus Creator2/1  "x"
  PS-Simulink Converter4/1 -> Bus Creator2/2  "y"
  PS-Simulink Converter11/1 -> Terminator6/1  "vz"
  connections:
  PS-Simulink Converter1/LConn1 -- MF Tire FL/RConn3
  PS-Simulink Converter/LConn1 -- MF Tire FL/RConn2
  Ground/RConn1 -- MF Tire FL/LConn1
  Transform Sensor-LocalBodyCS/RConn1 -- Rigid Transform/LConn1 -- MF Tire FL/RConn1 -- Rotation Axis Transform/RConn1 -- "Wheel "/RConn1
  Rim+Tire/RConn1 -- Geometry Transform/RConn1
  Geometry Transform/LConn1 -- Inertia/RConn1 -- Rotation Axis Transform/LConn1
  Transform Sensor-LocalBodyCS/LConn1 -- World Frame/RConn1 -- Transform Sensor-WorldCS/LConn1
  Transform Sensor-WorldCS/RConn1 -- Rigid Transform/RConn1
  Transform Sensor-WorldCS/RConn4 -- PS-Simulink Converter4/LConn1
  Transform Sensor-LocalBodyCS/RConn7 -- PS-Simulink Converter11/LConn1
  Transform Sensor-LocalBodyCS/RConn5 -- PS-Simulink Converter9/LConn1
  Transform Sensor-WorldCS/RConn2 -- PS-Simulink Converter2/LConn1
  Transform Sensor-WorldCS/RConn5 -- PS-Simulink Converter5/LConn1
  Transform Sensor-LocalBodyCS/RConn2 -- PS-Simulink Converter6/LConn1
  Transform Sensor-WorldCS/RConn3 -- PS-Simulink Converter3/LConn1
  Transform Sensor-LocalBodyCS/RConn3 -- PS-Simulink Converter7/LConn1
  Transform Sensor-LocalBodyCS/RConn4 -- PS-Simulink Converter8/LConn1
  Transform Sensor-LocalBodyCS/RConn6 -- PS-Simulink Converter10/LConn1

== system Tractor_Semitrailer_2023a/Tractor_semitrailer /Semitrailer/Trailer axle 2/Wheel FR ==
  Bus Creator : BusCreator  Inputs=6
  Bus Creator2 : BusCreator  Inputs=3
  Demux : Demux  Outputs=3
  Demux1 : Demux  Outputs=3
  Geometry Transform : sm_lib/Frames and Transforms/Rigid Transform  TranslationMethod=None  TranslationStandardOffset=0  TranslationStandardOffsetUnits=m  TranslationStandardAxis=+Y  TranslationCartesianOffset=[0 0 0]  TranslationCartesianOffsetUnits=m  TranslationROffset=0  TranslationROffsetUnits=m  TranslationZOffset=0  TranslationZOffsetUnits=m  TranslationThetaOffset=0  TranslationThetaOffsetUnits=deg  RotationMethod=StandardAxis  RotationAngleUnits=deg  RotationStandardAxis=+Z  RotationAngle=sideL*90  RotationArbitraryAxis=[0 0 1]  FollAlignAxisA=+X  BaseAlignAxisA=+Y  FollAlignAxisB=+Y  BaseAlignAxisB=+Z  RotationSequenceAxes=FollowerAxes  RotationSequence=XYX  RotationSequenceAngles=[0 0 0]  RotationSequenceAnglesUnits=deg  RotationMatrix=[1 0 0; 0 1 0; 0 0 1]  Quaternion=[1 0 0 0]
  Inertia : sm_lib/Body Elements/Inertia  InertiaType=Custom  Mass=wheelbody_mass  MassUnits=kg  CenterOfMass=[0 0 0]  CenterOfMassUnits=m  MomentsOfInertia=[Imat(1,1) Imat(2,2) Imat(3,3)]  MomentsOfInertiaUnits=kg*m^2  ProductsOfInertia=[0 0 0]  ProductsOfInertiaUnits=kg*m^2  GraphicType=None  MarkerShape=Inertia  MarkerSize=20  GraphicVisPropType=SimpleVisualProperties  GraphicDiffuseColor=[0.5 0.5 0.5]  GraphicSpecularColor=[0.5 0.5 0.5 1.0]  GraphicAmbientColor=[0.15 0.15 0.15 1.0]  GraphicEmissiveColor=[0.0 0.0 0.0 1.0]  GraphicShininess=75  GraphicOpacity=1.0
  MF Tire FL : sm_lib/Forces and Torques/Magic Formula Tire Force and Torque  TireSide=Right  TireParameters=tire_param  SlipMode=Combined  NumericParameters=[0.1 0.1 0.1 0.1 5.0 1e-4 1e-4 1e-7 1e-7 1e-4 1e-4 0.1 1e-4 1e-4 1e-4 1e-4 1e-4 1e-4 1e-4 1e-4 1e-4]  ScalingCoefficientLMUXMode=FromTireParameters  ScalingCoefficientLMUYMode=FromTireParameters  TireWrenchFrame=ContactFrame  SenseTireForce=on  SenseTireTorque=on  SensePneumaticTrail=off  SenseLongitudinalSlip=off  SenseSaturatedLongitudinalSlip=off  SenseSlipAngle=off  SenseSaturatedSlipAngle=off  SenseTurnSlip=off  SenseRelativeLongitudinalVelocity=off  SenseRelativeLateralVelocity=off  SenseLongitudinalSlipVelocity=off  SenseLateralSlipVelocity=off  SenseYawVelocity=off  SenseCamberAngle=off  SenseSaturatedCamberAngle=off  SenseCamberVelocity=off  SenseSpinVelocity=off  SenseFreeRadius=off  SenseLoadedRadius=off  SenseEffectiveRollingRadius=off  SenseLongitudinalFrictionCoefficient=off  SenseLateralFrictionCoefficient=off  SenseContactBaseRotation=off  SenseContactBaseTranslation=off  SenseContactFollowerRotation=off  SenseContactFollowerTranslation=off
  PS-Simulink Converter : nesl_utility/PS-Simulink Converter  PhysicalDomain=network_engine_domain  SubClassName=ps_output  LeftPortType=input  RightPortType=output  PseudoPeriodic=off  Frequencies=[]  VectorFormat=inherit  Unit=inherit  AffineConversion=off
  PS-Simulink Converter1 : nesl_utility/PS-Simulink Converter  PhysicalDomain=network_engine_domain  SubClassName=ps_output  LeftPortType=input  RightPortType=output  PseudoPeriodic=off  Frequencies=[]  VectorFormat=inherit  Unit=inherit  AffineConversion=off
  PS-Simulink Converter{2..11} (10 alike) : nesl_utility/PS-Simulink Converter  PhysicalDomain=network_engine_domain  SubClassName=ps_output  LeftPortType=input  RightPortType=output  PseudoPeriodic=off  Frequencies=[]  VectorFormat=1-D array  Unit=1  AffineConversion=off
  Reshape : Reshape
  Rigid Transform : sm_lib/Frames and Transforms/Rigid Transform  TranslationMethod=StandardAxis  TranslationStandardOffset=tire_width/2  TranslationStandardOffsetUnits=m  TranslationStandardAxis=-Z  TranslationCartesianOffset=[0 0 0]  TranslationCartesianOffsetUnits=m  TranslationROffset=0  TranslationROffsetUnits=m  TranslationZOffset=0  TranslationZOffsetUnits=m  TranslationThetaOffset=0  TranslationThetaOffsetUnits=deg  RotationMethod=None  RotationAngleUnits=deg  RotationStandardAxis=+Z  RotationAngle=0.0  RotationArbitraryAxis=[0 0 1]  FollAlignAxisA=+X  BaseAlignAxisA=+Y  FollAlignAxisB=+Y  BaseAlignAxisB=+Z  RotationSequenceAxes=FollowerAxes  RotationSequence=XYX  RotationSequenceAngles=[0 0 0]  RotationSequenceAnglesUnits=deg  RotationMatrix=[1 0 0; 0 1 0; 0 0 1]  Quaternion=[1 0 0 0]
  Rim+Tire : sm_lib/Body Elements/File Solid  ExtGeomFileName=wheel.STP  UnitType=Custom  ExtGeomFileUnits=mm  StepReaderType=HEX  ExportConvexHullGeometry=off  InertiaType=Custom  Mass=0  MassUnits=kg  CenterOfMass=[0 0 0]  CenterOfMassUnits=m  MomentsOfInertia=[0 0 0]  MomentsOfInertiaUnits=kg*m^2  ProductsOfInertia=[0 0 0]  ProductsOfInertiaUnits=kg*m^2  BasedOnType=Density  Density=1000  DensityUnits=kg/(m^3)  DoExposeReferenceFrame=on  SerializedFrames=<Frames/>  GraphicType=FromGeometry  MarkerShape=Sphere  MarkerSize=10  GraphicVisPropType=SimpleVisualProperties  GraphicDiffuseColor=[0.8 0.8 0.8]  GraphicSpecularColor=[0.5 0.5 0.5 1.0]  GraphicAmbientColor=[0.15 0.15 0.15 1.0]  GraphicEmissiveColor=[0.0 0.0 0.0 1.0]  GraphicShininess=75  GraphicOpacity=1.0
  Rotation Axis Transform : sm_lib/Frames and Transforms/Rigid Transform  TranslationMethod=None  TranslationStandardOffset=0  TranslationStandardOffsetUnits=m  TranslationStandardAxis=+Z  TranslationCartesianOffset=[0 0 0]  TranslationCartesianOffsetUnits=m  TranslationROffset=0  TranslationROffsetUnits=m  TranslationZOffset=0  TranslationZOffsetUnits=m  TranslationThetaOffset=0  TranslationThetaOffsetUnits=deg  RotationMethod=AlignedAxes  RotationAngleUnits=deg  RotationStandardAxis=-X  RotationAngle=0  RotationArbitraryAxis=[0 0 1]  FollAlignAxisA=+X  BaseAlignAxisA=+X  FollAlignAxisB=+Z  BaseAlignAxisB=+Y  RotationSequenceAxes=FollowerAxes  RotationSequence=XYX  RotationSequenceAngles=[0 0 0]  RotationSequenceAnglesUnits=deg  RotationMatrix=[1 0 0; 0 1 0; 0 0 1]  Quaternion=[1 0 0 0]
  Terminator{,1..6} (7 alike) : Terminator
  Transform Sensor-LocalBodyCS : sm_lib/Frames and Transforms/Transform Sensor  MeasurementFrame=NonRotatingFollower  RotationSequence=XYX  SenseAngle=off  SenseAxis=off  SenseQ=off  SenseR=off  SenseRotationSequence=off  SenseOmegaX=on  SenseOmegaY=on  SenseOmegaZ=on  SenseQDot=off  SenseRDot=off  SenseRotationSequenceDot=off  SenseAlphaX=off  SenseAlphaY=off  SenseAlphaZ=off  SenseQDDot=off  SenseRDDot=off  SenseX=off  SenseY=off  SenseZ=off  SenseRad=off  SenseAzim=off  SenseDist=off  SenseInc=off  SenseXDot=on  SenseYDot=on  SenseZDot=on  SenseRadDot=off  SenseAzimDot=off  SenseDistDot=off  SenseIncDot=off  SenseXDDot=off  SenseYDDot=off  SenseZDDot=off  SenseRadDDot=off  SenseAzimDDot=off  SenseDistDDot=off  SenseIncDDot=off
  Transform Sensor-WorldCS : sm_lib/Frames and Transforms/Transform Sensor  MeasurementFrame=World  RotationSequence=XYX  SenseAngle=off  SenseAxis=off  SenseQ=off  SenseR=on  SenseRotationSequence=off  SenseOmegaX=off  SenseOmegaY=off  SenseOmegaZ=off  SenseQDot=off  SenseRDot=off  SenseRotationSequenceDot=off  SenseAlphaX=off  SenseAlphaY=off  SenseAlphaZ=off  SenseQDDot=off  SenseRDDot=off  SenseX=on  SenseY=on  SenseZ=on  SenseRad=off  SenseAzim=off  SenseDist=off  SenseInc=off  SenseXDot=off  SenseYDot=off  SenseZDot=off  SenseRadDot=off  SenseAzimDot=off  SenseDistDot=off  SenseIncDot=off  SenseXDDot=off  SenseYDDot=off  SenseZDDot=off  SenseRadDDot=off  SenseAzimDDot=off  SenseDistDDot=off  SenseIncDDot=off
  World Frame : sm_lib/Frames and Transforms/World Frame
  "Wheel " : PMIOPort  Side=Left
  Ground : PMIOPort  Port=2  Side=Left
  Tire Foces : Outport
  Tire Position : Outport  Port=2
  wires:
  PS-Simulink Converter/1 -> Demux/1
  Demux/2 -> Bus Creator/2  "Lateral: Fy"
  Bus Creator/1 -> Tire Foces/1
  Demux/3 -> Bus Creator/3  "Normal: Fz"
  PS-Simulink Converter1/1 -> Demux1/1
  Demux1/2 -> Bus Creator/5  "Rolling Resistance: My"
  Demux1/3 -> Bus Creator/6  "Aligning: Mz"
  Demux1/1 -> Bus Creator/4  "Overturning: Mx"
  Demux/1 -> Bus Creator/1  "Longitudinal: Fx"
  PS-Simulink Converter6/1 -> Terminator1/1  "wx"
  PS-Simulink Converter10/1 -> Terminator5/1  "vy"
  PS-Simulink Converter8/1 -> Terminator3/1  "wz"
  PS-Simulink Converter2/1 -> Reshape/1
  PS-Simulink Converter9/1 -> Terminator4/1  "vx"
  PS-Simulink Converter5/1 -> Bus Creator2/3  "z"
  Bus Creator2/1 -> Tire Position/1
  PS-Simulink Converter7/1 -> Terminator2/1  "wy"
  Reshape/1 -> Terminator/1  "R"
  PS-Simulink Converter3/1 -> Bus Creator2/1  "x"
  PS-Simulink Converter4/1 -> Bus Creator2/2  "y"
  PS-Simulink Converter11/1 -> Terminator6/1  "vz"
  connections:
  PS-Simulink Converter1/LConn1 -- MF Tire FL/RConn3
  PS-Simulink Converter/LConn1 -- MF Tire FL/RConn2
  Ground/RConn1 -- MF Tire FL/LConn1
  Transform Sensor-LocalBodyCS/RConn1 -- "Wheel "/RConn1 -- Rotation Axis Transform/RConn1 -- MF Tire FL/RConn1 -- Rigid Transform/LConn1
  Rim+Tire/RConn1 -- Geometry Transform/RConn1
  Geometry Transform/LConn1 -- Inertia/RConn1 -- Rotation Axis Transform/LConn1
  Transform Sensor-LocalBodyCS/LConn1 -- World Frame/RConn1 -- Transform Sensor-WorldCS/LConn1
  Transform Sensor-WorldCS/RConn1 -- Rigid Transform/RConn1
  Transform Sensor-WorldCS/RConn4 -- PS-Simulink Converter4/LConn1
  Transform Sensor-LocalBodyCS/RConn7 -- PS-Simulink Converter11/LConn1
  Transform Sensor-LocalBodyCS/RConn5 -- PS-Simulink Converter9/LConn1
  Transform Sensor-WorldCS/RConn2 -- PS-Simulink Converter2/LConn1
  Transform Sensor-WorldCS/RConn5 -- PS-Simulink Converter5/LConn1
  Transform Sensor-LocalBodyCS/RConn2 -- PS-Simulink Converter6/LConn1
  Transform Sensor-WorldCS/RConn3 -- PS-Simulink Converter3/LConn1
  Transform Sensor-LocalBodyCS/RConn3 -- PS-Simulink Converter7/LConn1
  Transform Sensor-LocalBodyCS/RConn4 -- PS-Simulink Converter8/LConn1
  Transform Sensor-LocalBodyCS/RConn6 -- PS-Simulink Converter10/LConn1

== system Tractor_Semitrailer_2023a/Tractor_semitrailer /Semitrailer/Trailer axle 3/Brake//Wheel_bearing ==
  Mdrive : Inport
  Mbrake : Inport  Port=2
  Look-Up Table : Lookup  InputValues=[-5:0.05:5]  Table=-tanh(2*[-5:0.05:5])
  Product1 : Product  InputSameDT=on  SaturateOnIntegerOverflow=on  OutDataTypeStr=Inherit: Same as first input
  Rotational joint around y axis : Subsystem
  Sum : Sum  Inputs=++|
  axle : PMIOPort  Side=Left
  wheel : PMIOPort  Port=2  Side=Right
  omega : Outport  VectorParamsAs1DForOutWhenUnconnected=off
  wires:
  Mbrake/1 -> Product1/1
  Look-Up Table/1 -> Product1/2
  Product1/1 -> Sum/2
  Mdrive/1 -> Sum/1
  Rotational joint around y axis/1(Rotational speed) -> omega/1, Look-Up Table/1
  Sum/1 -> Rotational joint around y axis/1(Torque)
  connections:
  Rotational joint around y axis/LConn1 -- axle/RConn1
  wheel/RConn1 -- Rotational joint around y axis/RConn1

== system Tractor_Semitrailer_2023a/Tractor_semitrailer /Semitrailer/Trailer axle 3/Brake//Wheel_bearing1 ==
  Mdrive : Inport
  Mbrake : Inport  Port=2
  Look-Up Table : Lookup  InputValues=[-5:0.05:5]  Table=-tanh(2*[-5:0.05:5])
  Product1 : Product  InputSameDT=on  SaturateOnIntegerOverflow=on  OutDataTypeStr=Inherit: Same as first input
  Rotational joint around y axis : Subsystem
  Sum : Sum  Inputs=++|
  axle : PMIOPort  Side=Left
  wheel : PMIOPort  Port=2  Side=Right
  omega : Outport  VectorParamsAs1DForOutWhenUnconnected=off
  wires:
  Mbrake/1 -> Product1/1
  Look-Up Table/1 -> Product1/2
  Product1/1 -> Sum/2
  Mdrive/1 -> Sum/1
  Rotational joint around y axis/1(Rotational speed) -> omega/1, Look-Up Table/1
  Sum/1 -> Rotational joint around y axis/1(Torque)
  connections:
  Rotational joint around y axis/LConn1 -- axle/RConn1
  wheel/RConn1 -- Rotational joint around y axis/RConn1
